simulink model "powertrain"  (R2020b)
settings: Solver=FixedStepAuto  StartTime=0.0  StopTime=t(end)  RelTol=1e-3
PreLoadFcn:
  | C_sc = 1;
StartFcn:
  | C_sc = 1;
values from neighbouring files (symbols this model uses):
  D = 0    [model_fc.m]
  Ts = old_data.Ts    [model_fc.m]
undefined symbols (not defined in the file or in its folder): ANFIS, command, DiscIntNeverNeededParam, ECMS, Flight, in, Ion, Lithium, MPC, out, Tmpc, w
libraries: powerlib x25, neural x25, fuzblock x5, electricdrivelib x3, lib_converters x3, simulink x3, re_lib x1
(part 8 of 8)

== matlab function powertrain/EMS/Management Variant/MPC-1/PV - FC - control ==
  settings: updateMethod=DISCRETE  sampleTime=Ts
  data: Time input; Vdc_command input; Vfc input; Ifc_in input; Vbatt input; Ibatt_in input; Vpv input; Ifc output; Vfc_conv output; IO_fc_conv output; Pload input; Ipv_in input; SOC input; Ipv output; Vpv_conv output; IO_pv_conv output; Ipvout input; Vdc_real input; Pout_real input; Control_pv output; IO_pv_conv_value input; IO_fc_conv_value input; Control_pv_choose_var input
function [Ifc,Vfc_conv,IO_fc_conv,Ipv,Vpv_conv,IO_pv_conv,Control_pv] = fcn(Time, Vdc_command,Vfc,Ifc_in, Vbatt, Ibatt_in, Vpv, Pload, Ipv_in, SOC, Ipvout, Vdc_real, Pout_real, IO_pv_conv_value, IO_fc_conv_value, Control_pv_choose_var)
    
    
    %% Test for pv panel P&O algo
    persistent Ppv_pre Ppv_w_pre;
    dataType = 'double';
    
    if isempty(Ppv_pre)
        Ppv_pre=0;
        Ppv_w_pre = 200;
    end
    
    if Control_pv_choose_var == 0 % Auto
        Control_pv = 2; % 1 = MPPT | 2 = Cascade Control
    else
        Control_pv = Control_pv_choose_var;
    end
    
    % ?? utile pour le début mais ne fonctionne pas après
%         if Pload == 0 && Control_pv_choose_var == 0
%             Control_pv = 1;
%         end
    
    
    
    Ppv_out = Ipvout*Vdc_real;
    Ppv_in = Ipv_in*Vpv;
    Delta_PV = 0.5;
    Ppv_wanted = Ppv_in;
    
    if Control_pv == 2 % Cascade control
        if mod(Time,2e-4) == 0
            if Ppv_in < Ppv_pre
                Ppv_wanted  = Ppv_in - Delta_PV;
            end
            if Ppv_in > Ppv_pre
                Ppv_wanted  = Ppv_in + Delta_PV;
            end
        end
        if Ppv_out < 0
            Ppv_wanted = 180;
        end
        
        Ipv = Ppv_wanted/Vpv;
    else
        Ipv = 0;
    end
%         Ipv = 180/Vpv;
    Vpv_conv = Vdc_command;
    
    
    % PV converter operates ?
    IO_pv_conv = IO_pv_conv_value;
    
    Ppv_pre = Ppv_in;
    Ppv_w_pre = Ppv_wanted;
    
    
    %% Set if needed
    %     Ipv = 185/Vpv;
    
    
    %% Set max current wanted for the fuel cell
    %     Ifc = 200/Vfc; % doesn't work with my own model
    %     Ifc = 7; % doesn't work with battery ??
    Ifc = 1100/Vfc; % work now ??

    Vfc_conv = Vdc_command;
    if Ifc_in < Ifc
        Vfc_conv = 100;
    end

    
    % FC converter operates ?
    IO_fc_conv = IO_fc_conv_value;
    
end

== matlab function powertrain/EMS/Management Variant/ANFIS-ECMS/MATLAB Function ==
  settings: updateMethod=DISCRETE  sampleTime=Ts
  data: Vbatt input; Ibatt input; Ibatt_out input; Ibatt_1 output; Ifc_out input; Vpv input; Ipv input; Ipv_out input; Pload input; Vdc input; Vdc_wanted input; Pout input; Ibatt_2 output; Ibatt_3 output; IO_batt_conv output; IO_batt_conv_value input; Ifc_boost input; Vfc input
function [Ibatt_1, Ibatt_2, Ibatt_3,  IO_batt_conv] = fcn(Vbatt, Ibatt,Ibatt_out, Ifc_out, Vpv, Ipv, Ipv_out,Pload,Vdc,Vdc_wanted, Pout, IO_batt_conv_value, Ifc_boost, Vfc)
    %% Part - 1
    %     FC = Vfc * Ifc_boost;
    %     FC = Vfc * Ifc_in;
    %     FC = Vdc_wanted * Ifc_out;
    FC = Vdc * Ifc_out;
    
    %     PV = Vpv * Ipv_boost;
%         PV = Vpv * Ipv; % stable pv panel but not good
    %     PV = Vdc_wanted * Ipv_out;
    PV = Vdc * Ipv_out; % marche mieux avec celui ci mais pv pas au max
    
    %     Batt = Vbatt * Ibatt;
    Batt = Vdc * Ibatt_out/0.9;
    
    %     Ibatt_1 = (Pload - FC - PV)/Vdc_wanted;
    %     Ibatt_1 = (Pload - FC - PV)/Vdc;
    Ibatt_1 = (Pload - FC - PV - Batt)/Vdc;
    %     Ibatt_1 = -10;
    
    %% Part - 2
    Ibatt_2 = Pload - Pout;
    
    %% Part - 3
    Ibatt_3 = Vdc_wanted - Vdc;
    
    %% Activate conv
    IO_batt_conv = IO_batt_conv_value;
end

== matlab function powertrain/EMS/Management Variant/ANFIS-ECMS/MATLAB Function1 ==
  settings: updateMethod=DISCRETE  sampleTime=Ts
  data: current_comm input; conv output; Pload input; Vbus_required input; current_command output; V_batt_conv output; DV input
function [conv, current_command,V_batt_conv] = fcn(current_comm, Pload, Vbus_required, DV)
    if current_comm < 0
        conv = 1;
        V_batt_conv = Vbus_required; % (55)
    else
        conv = 0;
        V_batt_conv = Vbus_required;
    end
%     V_batt_conv = 120;
    current_command = current_comm;
    Vbatt_conv = V_batt_conv + DV;
end

%     if Pload == 0 || current_comm < 0
%         conv = 1;
%         V_batt_conv = 50;
%     else
%         conv = 0;
%         V_batt_conv = Vbus_required;
%     end
%     current_command = current_comm;

== matlab function powertrain/PEMFC matfunc V3 - multi/MATLAB Function ==
  settings: updateMethod=DISCRETE  sampleTime=Ts
  data: U_H2 output; U_O2 output; R_ohm output; Ifc input; E_Ner output; E_ohm output; E_con output; E_act_steady output; E_act input; E_act_d output; limit output
function [U_H2,U_O2,R_ohm,E_Ner,E_ohm,E_con,E_act_steady,E_act_d,limit] = fcn(Ifc,E_act)
%     https://link.springer.com/article/10.1007/s40565-016-0196-5
%     Modeling and Simulation of a Proton Exchange Membrane Fuel Cell Alongside a Waste Heat Recovery System Based on the Organic Rankine Cycle in MATLAB/SIMULINK Environment
%     MATHEMATICAL MODELLING FOR PROTON EXCHANGE MEMBRANE FUEL CELL (PEMFC) 
%     https://www.scirp.org/pdf/epe_2020112310053180.pdf#page=17&zoom=100,72,604
%     H-Series Fuel Cell Stacks

    %% constants:
    R = 8.3145;
    Pstd = 101325;
    nF = 2*96485;
    C_act = 2;
    A = 19.6*4.0;
    T = 303.15;
    Nfc = 50;
    lambda = 14;
    l = 21e-4 * 10^-2;
%     l = 1.27e-4;
    
    J = Ifc/A;
    JM = 45/A;
    Pa = 1.45;
    Pc = 1;
    Tc = T-273.15;
    coeff = 1;
        
%     if Ifc <=0
%         Ifc = 40;
%     end
    
    PH2Osat = 10^(-2.18+2.95e-2*Tc-9.18e-5*Tc^2+1.44e-7*Tc^3);
    
    P_H2 = 0.5*PH2Osat*(exp(-(1.635*J/T^1.334))*(Pa/PH2Osat)-1);
    P_O2 = PH2Osat*(exp(-(4.192*J/T^1.334))*(Pc/PH2Osat)-1);
    

    %% Saturation at start
    if -1.87e-4*log(Ifc) > 0
        k = 0;
    else
        if -1.87e-4*log(Ifc) < -1.2
            k = -1.2;
        else
            k = -1.87e-4*log(Ifc);
        end
    end
    %% Nernst Voltage
    E_Ner = 1.229 + (T-298.15) * (-0.85e-3) + T*R/nF * log(P_H2*P_O2^0.5);
    
    %% Activation loss
    % Pressure not in Pa ?
    CO2 = (P_O2/(5.08e6))*exp(498/T);
    CH2 = (P_H2/(1.09e6))*exp(-77/T);
    E_act_steady=-0.9514 + T * (2.86e-3+2e-4*log(200)+4.3e-5*log(CH2)+7.4e-5*log(CO2)+k);
%     E_act_steady = -0.9514 + 3.12e-3*T + 7.4e-5*T*log(CO2) -1.87e-4*T*log(Ifc);
    
    %% Ohmic loss
    E_ohm = - Ifc*(l/((lambda*5.139e-3-3.26e-3)*exp(1268*(1/303-1/T))));
    R_ohm = (l/((lambda*5.139e-3-3.26e-3)*exp(1268*(1/303-1/T))));
    
    %% Concentration loss
%     if T>= 312.15
%         E_con = (1.1e-4-1.2e-6*(T-273.15))*exp(8*Ifc/40);
%     else
%         E_con = (3.3e-3-8.2e-5*(T-273.15))*exp(8*Ifc/40);
%     end

%     E_con = 3*R*T/(2*nF)*log(1-J/JM)-1.5607*R*T/(2*nF);
        if J/JM < 1
        E_con = 3*R*T/(2*nF)*log(1-J/JM)-1.5607*R*T/(2*nF);
    else
%         E_con = -abs(3*R*T/(2*nF)*log(complex(1-J/(JM-0.001)))-1.5607*R*T/(2*nF));
        E_con = 3*R*T/(2*nF)*log(J/JM)-1.5607*R*T/(2*nF);
    end
    
    %% with coefficient
    E_con = coeff * E_con;
    E_act_steady = coeff * E_act_steady;
    E_ohm = coeff * E_ohm;
    E_Ner = coeff * E_Ner;
    
        
    %% activation dynamic loss:
    below = -E_act_steady-E_con;
    E_act_d = (Ifc/C_act)*(1-E_act/below);
%     E_act_d = 0;

    %% Fuel utilization
    U_H2 = 60000*Ifc*R*T*Nfc/(nF*1.16*1*0.9995*Pstd);
    
    %% Air utilization
    U_O2 = 60000*Ifc*R*T*Nfc/(2*nF*0.0181*1*0.21*Pstd);
    limit = 1;
    if J/JM >= 1
            E_con = 0;
            E_act_steady = 0;
            E_ohm = 0;
            E_act_d = 0;
            E_Ner = -35*Ifc;
            if E_Ner <= 0
                E_Ner = 0;
            end
            limit = 0;
    end
    
    
    %%
end

== matlab function powertrain/MATLAB Function ==
  settings: updateMethod=DISCRETE  sampleTime=Ts
  data: ep output; ev output; time input; error_power output; Prequired input; Preal input; Vbus_required input; Vbus_real input; error_voltage output
function [ep,ev,error_power, error_voltage] = fcn(time, Prequired, Preal, Vbus_required, Vbus_real)
    ep = (Preal-Prequired)^2;
    ev = (Vbus_real-Vbus_required)^2;
    
    error_power = 100*abs(Preal-Prequired)/abs(Prequired);
    error_voltage = 100*abs(Vbus_real-Vbus_required)/Vbus_required;
end

== matlab function powertrain/EMS/Management Variant/ANFIS-ECMS/PV - FC - control1 ==
  settings: updateMethod=DISCRETE  sampleTime=Ts
  data: Time input; Vdc_command input; Vfc input; Ifc_in input; Vbatt input; Ibatt_in input; Vpv input; Ifc output; Vfc_conv output; IO_fc_conv output; Pload input; Ipv_in input; SOC input; Ipv output; Vpv_conv output; IO_pv_conv output; Ipvout input; Vdc_real input; Pout_real input; Control_pv output; IO_pv_conv_value input; IO_fc_conv_value input; Control_pv_choose_var input; fuzzy_out input; NNres input
function [Ifc,Vfc_conv,IO_fc_conv,Ipv,Vpv_conv,IO_pv_conv,Control_pv] ...
        = fcn(Time, Vdc_command,Vfc,Ifc_in, Vbatt, Ibatt_in, Vpv, Pload,...
        Ipv_in, SOC, Ipvout, Vdc_real, Pout_real, IO_pv_conv_value,...
        IO_fc_conv_value, Control_pv_choose_var, fuzzy_out, NNres)
    
    
    %% PV - Test for pv panel algo in Cascade control
    persistent Ppv_pre Ppv_w_pre;
    dataType = 'double';
    
    if isempty(Ppv_pre)
        Ppv_pre=0;
        Ppv_w_pre = 200;
    end
    
    if Control_pv_choose_var == 0 % Auto
        Control_pv = 2; % 1 = MPPT | 2 = Cascade Control
    else
        Control_pv = Control_pv_choose_var;
    end
    
    % ?? utile pour le début mais ne fonctionne pas après
%         if Pload == 0 && Control_pv_choose_var == 0
%             Control_pv = 1;
%         end
    
    
    
    Ppv_out = Ipvout*Vdc_real;
    Ppv_in = Ipv_in*Vpv;
    Delta_PV = 0.5;
    Ppv_wanted = Ppv_in;
    
    if Control_pv == 2 % Cascade control
        if mod(Time,2e-4) == 0
            if Ppv_in < Ppv_pre
                Ppv_wanted  = Ppv_in - Delta_PV;
            end
            if Ppv_in > Ppv_pre
                Ppv_wanted  = Ppv_in + Delta_PV;
            end
        end
        if Ppv_out < 0
            Ppv_wanted = 180;
        end
        
        Ipv = Ppv_wanted/Vpv;
    else
        Ipv = 0;
    end
    Vpv_conv = Vdc_command;
    
    
    % PV converter operates ?
    IO_pv_conv = IO_pv_conv_value;
    
    Ppv_pre = Ppv_in;
    Ppv_w_pre = Ppv_wanted;
    
    
    
    %% Set current for the FC
    Ifc = fuzzy_out(NNres) * 1100/Vfc;
    

    Vfc_conv = Vdc_command;
    if Ifc_in < Ifc && (Vdc_real > Vdc_command*0.97 || Vdc_real < Vdc_command * 1.03)
        Vfc_conv = 100;
    end
       
    
    % FC converter operates ?
    IO_fc_conv = IO_fc_conv_value;
    
end

== matlab function powertrain/EMS/Management Variant/ECAEMS/MATLAB Function ==
  settings: updateMethod=DISCRETE  sampleTime=Ts
  data: Vbatt input; Ibatt input; Ibatt_out input; Ibatt_1 output; Ifc_out input; Vpv input; Ipv input; Ipv_out input; Pload input; Vdc input; Vdc_wanted input; Pout input; Ibatt_2 output; Ibatt_3 output; IO_batt_conv output; IO_batt_conv_value input; Ifc_boost input; Vfc input
function [Ibatt_1, Ibatt_2, Ibatt_3,  IO_batt_conv] = fcn(Vbatt, Ibatt,Ibatt_out, Ifc_out, Vpv, Ipv, Ipv_out,Pload,Vdc,Vdc_wanted, Pout, IO_batt_conv_value, Ifc_boost, Vfc)
    %% Part - 1
    %     FC = Vfc * Ifc_boost;
    %     FC = Vfc * Ifc_in;
    %     FC = Vdc_wanted * Ifc_out;
    FC = Vdc * Ifc_out;
    
    %     PV = Vpv * Ipv_boost;
%         PV = Vpv * Ipv; % stable pv panel but not good
    %     PV = Vdc_wanted * Ipv_out;
    PV = Vdc * Ipv_out; % marche mieux avec celui ci mais pv pas au max
    
    %     Batt = Vbatt * Ibatt;
    Batt = Vdc * Ibatt_out;
    
    %     Ibatt_1 = (Pload - FC - PV)/Vdc_wanted;
    %     Ibatt_1 = (Pload - FC - PV)/Vdc;
    Ibatt_1 = (Pload - FC - PV - Batt)/Vdc;
    %     Ibatt_1 = -10;
    
    %% Part - 2
    Ibatt_2 = Pload - Pout;
    
    %% Part - 3
    Ibatt_3 = Vdc_wanted - Vdc;
    
    %% Activate conv
    IO_batt_conv = IO_batt_conv_value;
end

== matlab function powertrain/EMS/Management Variant/MPC-1/MATLAB Function2 ==
  settings: updateMethod=DISCRETE  sampleTime=Ts
  data: Vin input; Vin output; Iin output; Iin input; Vdc input; Ifc_out input; Vdc_ref input; ILmax input; time_data input; old_E_act_d input; old_lim input; sampleTime input; Pin output; Vout output; Iout output; Pout output; Ifc_boost output; Tmpc input; IO_fc_conv input; IO_pv_conv input; Control_pv_choose_var input; Vfc_conv output; IO_fc output; Ipv output; Vpv_conv output; IO_pv output; Control_pv output; Pload input; SOC input; Pload_est input; Vdc_command input; Ipv_out input; Pout_real input
function [Vin, Iin, Pin, Vout, Iout, Pout, Ifc_boost, Vfc_conv, IO_fc, ...
        Ipv, Vpv_conv, IO_pv, Control_pv] = test(Vin, Iin, Vdc, Ifc_out,...
        Vdc_ref, ILmax, time_data, old_E_act_d, old_lim, sampleTime,Tmpc, ...
        IO_fc_conv,IO_pv_conv,Control_pv_choose_var, Pload, SOC, ...,
        Pload_est, Vdc_command,Ipv_out, Pout_real)
    
    coder.extrinsic('evalin');
    coder.extrinsic('GlobalSearch');
    coder.extrinsic('createOptimProblem');
    coder.extrinsic('opti_fcn');
    coder.extrinsic('assignin')
    %% init
    persistent data Pfc_command_pre Pload_full Tsss
    
    if isempty(data)
        Pfc_command_pre = 250;
        
        
        
        Pload_full = evalin('base', 'w');
        data = struct;
        %% variables / states
        data.x_k= [-0.014465353509422;72];
        %         [Iin;Vdc];
        data.e_pre = 0;
        data.e2_pre = 0;
        data.pi_pi = 0;
        data.pi_ii = 0;
        data.E_act = 0;
        data.old_E_act_bl = 0;
        data.old_E_act_d = 0;
        data.old_lim = 0;
        data.Efc = Vin;
        
        %% static data
        data.Ts = sampleTime;
        % converter data
        data.L = 2e-3;
        L = 2e-3;
        data.Ca = 1e-4;
        Ca = 1e-4;
        data.Cdc = 1;
        Cdc = 1;
        
        % regulators data
        data.Ct = Ca + Cdc;
        Ct = Ca + Cdc;
        
        T_v_bst = 1;
        T_i_bst = 1;
        damp = 0.707;
        % Current regulator
        zetai=damp;
        thau_si=T_i_bst/10;
        zetawni=(-log(0.05*sqrt(1-zetai^2)))/thau_si;
        data.Kpi=2*L*zetawni / 1000;
        wni=zetawni/zetai;
        data.Kii=L*wni^2 / 1000;
        
        % Voltage regulator
        zetav=damp;
        thau_sv=T_v_bst; %response time
        zetawnv=(-log(0.05*sqrt(1-zetav^2)))/thau_sv;
        data.Kpv=2*Ct*zetawnv;
        wnv=zetawnv/zetav;
        data.Kiv=Ct*wnv^2;
        
        % fuel cell data
        data.Ncell = 50;
        data.eff = 0.9;
        data.T = 303.15;
        data.Rohm = 0.061871;
        data.R_ = 8.3145;
        data.Pstd = 101325;
        data.nF = 2*96485;
        data.C_act = 2;
        A = 19.6*4.0;
        data.A = 19.6*4.0;
        data.Nfc = 50;
        data.lambda = 14;
        data.l = 21e-4 * 10^-2;
        data.JM = 45/A;
        data.Pa = 1.45;
        data.Pc = 1;
        data.coeff = 1;
        Tsss = evalin('base', 'Ts');
    end
    Ts = 1e-3;
    Hp = 20;
    TsOpti = Ts*1e3;
    
    %     Ts = 1e-3; %     Hp = 20; %     TsOpti = Ts*1e3;
    
    
    if Control_pv_choose_var == 0 % Auto
        Control_pv = 2; % 1 = MPPT | 2 = Cascade Control
    else
        Control_pv = Control_pv_choose_var;
    end
    
    IO_pv = IO_pv_conv;
    Vpv_conv = 72;
    Ipv = 0;
    
    
    
    %% approximation of states of the FC part
    %     data.old_E_act_d = old_E_act_d;
    %     data.old_lim = old_lim;
    
    %     data.x_k = [Iin;Vdc];
    
    %     data.Ts = Ts;
    [Vin,Vout,Iout,Pin,Pout,data] = res_fun(Vdc,Ifc_out,ILmax,Vdc_ref,data);
    
    Iin = data.x_k(1);
    Vout = data.x_k(2);
    
    %% FC control
    % FC converter operates ?
    IO_fc = IO_fc_conv;
    
    currind = time_data/Ts;
    
    %     Pload_est = Pload_full(time_data(1)/Ts)
    %     Pload_est = Pload_full(currtime(1:Hp));
    %%%%%%%%
    %%%     ECMS algo:
    %         if (false)
    len = 0;
    len = length(Pload_full);
    if mod((time_data/TsOpti),Hp/2) == 1 && len(1)-currind > TsOpti/Ts*Hp
        SOC_min=40; SOC_max=90;
        Ppv_out = Ipv_out*Vdc;
%         if Pout_real-Ppv_out > 0 || SOC < SOC_min
%             Pfc_command_min=150;
%         else
%             Pfc_command_min = 0;
%         end
        Pfc_command_min=150;
        Pfc_command_max=1100;
        
        size_step = 0:TsOpti/Ts:TsOpti/Ts*Hp;
        currtime = round(currind+size_step);
        Pload_est = Pload_full(currtime(1:Hp));
%         Pload_est = Pload_est - Ppv_out;
        %         Pload_est = sum(Pload_est) - Ppv_out*Hp;
        
        
        
        %define Matrix Aeq
        
        %         Aeq=[0 1];
        %         Aeq=[0 1];
        
        %define Matrix beq
        mu=0.6;
        %         beq=[1-2*mu*((SOC-0.5*(SOC_max+SOC_min))/(SOC_max+SOC_min))];
        k=1-2*mu*((SOC-0.5*(SOC_max+SOC_min))/(SOC_max+SOC_min));
        %     beq=[1-2*mu*((SOC-0.5*(SOC_max+SOC_min))/(SOC_max+SOC_min)); Pload-Ppv_out];
        
        %         %define boundary conditions
        %         lb=[Pfc_command_min, 0];
        %         ub=[Pfc_command_max, 100];
        %
        %         %define initial conditions
        %         x0=[100, 0.1];
        %define boundary conditions
        lb=[Pfc_command_min];
        ub=[Pfc_command_max];
        
        %define initial conditions
        x0=[Pfc_command_pre];
        
        
        %         Pfc_command_pre
        Vdc_real = data.x_k(2);
        Ifc_out = Pout/Vdc_real;
        %         options = optimoptions('fmincon','Algorithm','sqp',...
        %             'Display','off','MaxFunctionEvaluations',500,'MaxIterations',300,...
        %             'DiffMinChange',10);
        %         [y,fval] = fmincon(@(x)loop_res_fun(x,Vin,Vdc,Ifc_out,ILmax,Vdc_ref,data,Hp,Pload_est,k),x0,[],[],[],[],lb,ub,[],options);
        
        Ifc_boost = zeros(1,1);
        y = opti_fcn(x0,lb,ub,Vin,Vdc,Ifc_out,ILmax,Vdc_ref,data,Hp,Pload_est,Ppv_out,k,TsOpti);
        
        Pfc=y(1);
        %         alpha=y(2);
        
        
        %         Pfc = 1100;
    else
        Pfc = Pfc_command_pre;
    end
    Pfc_command_pre = Pfc;
    %%%%%%%%
    
    
    
    Ifc_boost = Pfc/Vin;
    
    % Converter command output voltage
    Vfc_conv = Vdc_command;
    if Iin < Ifc_boost
        %     if Iin < 0.9*Ifc_boost || Iin > 1.1*Ifc_boost
        Vfc_conv = 100;
    end
    
end

% non linear constraints if needed :
% https://fr.mathworks.com/matlabcentral/answers/102632-what-is-the-calling-order-of-the-objective-function-and-nonlinear-constraint-function-for-optimizati

function f = loop_res_fun(x,Vin,Vdc,Ifc_out,ILmax,Vdc_ref,data,Hp,Pload_est,k)
    %     coder.extrinsic('res_fun');
    Ptot_fc = 0;
    err = 0;
    for i=1:Hp
        ILmax = x(1) / Vin;
        Vdc_real = data.x_k(2);
        [Vin,Vout,Iout,Pin,Pout,data] = res_fun(Vdc_real,Ifc_out,ILmax,Vdc_ref,data);
        Vdc_real = data.x_k(2);
        Ifc_out = Pout/Vdc_real;
        if data.x_k(1) > ILmax
            Vdc_ref = 100;
        else
            Vdc_ref = 72;
        end
        Ptot_fc = Ptot_fc + Pin;
        %         if Pload_est(i) - Pout > 850 || Pload_est(i) - Pout < -150
        %             err = err + 1000;
        %         end
    end
    %     f = Hp*data.Ts * (Ptot_fc*(1-x(2)) + x(2)*sum(Pload_est) + err)
    f = Hp*data.Ts * (Ptot_fc*(1-k) + k*sum(Pload_est) + err)
    x
    x-100
    
    
end

function [Vin,Vout,Iout,Pin,Pout,new_data] = res_fun(Vdc,Ifc_out,ILmax,Vdc_ref,data)
    %% get data
    Ts = data.Ts;
    % converter data
    L = data.L;
    Ca = data.Ca;
    
    % Current regulator
    Kpi = data.Kpi;
    Kii = data.Kii;
    
    % Voltage regulator
    Kpv = data.Kpv;
    Kiv = data.Kiv;
    
    % fuel cell data
    Ncell = data.Ncell;
    eff = data.eff;
    T = data.T;
    Rohm = data.Rohm;
    R_ = data.R_;
    Pstd = data.Pstd;
    nF = data.nF;
    C_act = data.C_act;
    Nfc = data.Nfc;
    lambda = data.lambda;
    l = data.l;
    JM = data.JM;
    Pa = data.Pa;
    Pc = data.Pc;
    coeff = data.coeff;
    
    
    
    % states
    %     x_k=[Iin;Vdc];
    x_k=data.x_k;
    e_pre=data.e_pre;
    e2_pre=data.e2_pre;
    pi_pi=data.pi_pi;
    pi_ii=data.pi_ii;
    E_act=data.E_act;
    old_E_act_bl=data.old_E_act_bl;
    old_E_act_d=data.old_E_act_d;
    old_lim=data.old_lim;
    Efc=data.Efc;
    
    
    %% start the function
    R = Vdc/Ifc_out;
    x_k(2) = Vdc; %%%%%%%%%%%% changed here
    
    
    
    % Vdc_ref = given by EMS
    % ILmax = given by EMS
    
    %     if x_k(1)<0.001
    %         x_k(1) = 0.001;
    %     end
    
    
    %     Vin = Efc - Rohm * x_k(1);
    Vin = Efc;
    if Vin <= 0
        Vin = 60.484318707027604;
    end
    
    
    %% BOOST PART
    % control part voltage:
    e=(Vdc_ref - x_k(2));
    %     e=(Vdc_ref - Vdc_real);
    pi_pi = min(0.5,max(-0.5,pi_pi + Kiv*Ts*e_pre)); % sat:[-0.5; 0.5]
    out_pi_1 = min(0.5,max(-0.5,Kpv*e + pi_pi)); % sat:[-0.5; 0.5]
    
    sub = max(0.01,eff*Vin); % sat:[0.01; Inf]
    %     temp = min(ILmax,max(0,(out_pi_1+x_k(2)/R)*x_k(2)/sub)); % sat:[0; ILmax]
    temp = min(ILmax,max(0,(out_pi_1+x_k(2)*(1/(5e3)+1/R))*x_k(2)/sub)); % sat:[0; ILmax]
    %     temp = (out_pi_1+Vdc_real/R)*Vdc_real/sub;
    
    
    % control part current
    e2 = temp - x_k(1);
    %     e2 = temp - iL;
    pi_ii = min(50,max(-50,pi_ii + Kii*Ts*e2_pre)); % sat:[-50; 50]
    out_pi_2 = min(50,max(-50,Kpi*e2 + pi_ii)); % sat:[-50; 50]
    
    sub_2 = max(0.01,x_k(2)); % sat:[0.01; Inf]
    %     sub_2 = max(0.01,Vdc_real);
    d = min(1,max(0,1-(Vin-out_pi_2)/sub_2)); % sat:[0; 1]
    
    
    
    A = [-0.002/L -(1-d)/L;(1-d)*eff/Ca*R/(R+0.002) -1/((R+0.002)*Ca)];
    B = [1/L; 0];
    C = [1 0];
    D = 0;
    
    % continuous to discrete (exact)
    %     Ai = expm(Ts*A);
    %     Bi = inv(A)*(Ai - eye(2))*B;
    
    % approx : (https://en.wikipedia.org/wiki/Discretization)
    Ai = eye(2)+A*Ts;
    Bi = Ts*B;
    
    x_k1 = Ai*x_k+Bi*Vin;
    y = C*x_k;
    
    
    %% Outputs
    x_k = x_k1;
    %     x_k(2) = Vdc_real;
    %     x_k(1) = iL;
    %     if x_k(1) < 0.001
    %         x_k(1) = 0.001;
    %     end
    
    Vout = x_k(2);
    Rreal = R+0.002;
    Iout_1 = Vout/Rreal;
    Iout = (Iout_1 - Vout/(5e3));
    
    % works well
    Vout = 72;
    x_k(2) = Vout;
    
    %     x_k(2) = Vdc;
    Iout = Vout/R;
    
    
    Pin = min(2000,max(-100,  Vin*x_k(1))); % sat:[-100; 2000]
    
    Pout = min(2000,max(-500, Vout*Iout));  % sat:[-500; 2000]
    %     Pout = min(2000,max(-500, 0.9*Pin));  % sat:[-500; 2000]
    
    
    
    %% FC PART
    if x_k(1)<0.001
        x_k(1) = 0.001;
    end
    if x_k(1)>100
        x_k(1) = 100;
    end
    Ifc = x_k(1);
    
    J = Ifc/data.A;
    Tc = T-273.15;
    
    PH2Osat = 10^(-2.18+2.95e-2*Tc-9.18e-5*Tc^2+1.44e-7*Tc^3);
    
    P_H2 = 0.5*PH2Osat*(exp(-(1.635*J/T^1.334))*(Pa/PH2Osat)-1);
    P_O2 = PH2Osat*(exp(-(4.192*J/T^1.334))*(Pc/PH2Osat)-1);
    
    
    % Saturation at start
    if -1.87e-4*log(Ifc) > 0
        k = 0;
    else
        if -1.87e-4*log(Ifc) < -1.2
            k = -1.2;
        else
            k = -1.87e-4*log(Ifc);
        end
    end
    
    % Nernst Voltage
    E_Ner = 1.229 + (T-298.15) * (-0.85e-3) + T*R_/nF * log(P_H2*P_O2^0.5);
    
    % Activation loss
    % Pressure not in Pa ?
    CO2 = (P_O2/(5.08e6))*exp(498/T);
    CH2 = (P_H2/(1.09e6))*exp(-77/T);
    E_act_steady=-0.9514 + T * (2.86e-3+2e-4*log(200)+4.3e-5*log(CH2)+7.4e-5*log(CO2)+k);
    %     E_act_steady = -0.9514 + 3.12e-3*T + 7.4e-5*T*log(CO2) -1.87e-4*T*log(Ifc);
    
    % Ohmic loss
    E_ohm = - Ifc*(l/((lambda*5.139e-3-3.26e-3)*exp(1268*(1/303-1/T))));
    R_ohm = (l/((lambda*5.139e-3-3.26e-3)*exp(1268*(1/303-1/T))));
    
    % Concentration loss
    %     if T>= 312.15
    %         E_con = (1.1e-4-1.2e-6*(T-273.15))*exp(8*Ifc/40);
    %     else
    %         E_con = (3.3e-3-8.2e-5*(T-273.15))*exp(8*Ifc/40);
    %     end
    
    if J/JM < 1
        E_con = 3*R_*T/(2*nF)*log(1-J/JM)-1.5607*R_*T/(2*nF);
    else
        %         E_con = -abs(3*R*T/(2*nF)*log(complex(1-J/(JM-0.001)))-1.5607*R*T/(2*nF));
        E_con = 3*R_*T/(2*nF)*log(J/JM)-1.5607*R_*T/(2*nF);
    end
    
    % with coefficient
    E_con = coeff * E_con;
    E_act_steady = coeff * E_act_steady;
    E_ohm = coeff * E_ohm;
    E_Ner = coeff * E_Ner;
    
    
    % activation dynamic loss:
    below = -E_act_steady-E_con;
    E_act_d = (Ifc/C_act)*(1-E_act/below);
    
    % Fuel utilization
    U_H2 = 60000*Ifc*R_*T*Nfc/(nF*1.16*1*0.9995*Pstd);
    
    % Air utilization
    U_O2 = 60000*Ifc*R_*T*Nfc/(2*nF*0.0181*1*0.21*Pstd);
    limit = 1;
    if J/JM >= 1
        E_con = 0;
        E_act_steady = 0;
        E_ohm = 0;
        E_act_d = 0;
        E_Ner = -35*Ifc;
        if E_Ner <= 0
            E_Ner = 0;
        end
        limit = 0;
    end
    
    
    % Efc
    %     E_act_bl =  (old_E_act_bl + Ts*old_E_act_d);
    E_act_bl =  (old_E_act_bl + Ts*E_act_d);
    old_E_act_d = E_act_d;
    E_act = old_lim *E_act_bl;
    old_lim = limit;
    old_E_act_bl = E_act_bl;
    
%     E_act_bl =  (old_E_act_bl + Ts*old_E_act_d);
%     old_E_act_d = E_act_d;
%     old_E_act_bl = E_act_bl;
%     E_act = old_lim *E_act_bl;
%     old_lim = limit;
    
    old_lim = limit;
    
    Efc = Ncell*(E_Ner + E_ohm + E_con - E_act)-Rohm*x_k(1);
    if Efc <= 0
        Efc = 0;
    end
    %     Vin = Efc;
    Iin = x_k(1);
    
    %% save states + data
    
    data.x_k= x_k;
    data.e_pre =e;
    data.e2_pre = e2;
    data.pi_pi = pi_pi ;
    data.pi_ii = pi_ii ;
    data.E_act = E_act ;
    data.old_E_act_bl = old_E_act_bl ;
    data.old_E_act_d = old_E_act_d;
    data.old_lim = old_lim ;
    data.Efc = Efc;
    
    
    new_data = data;
    
    
    %% compute the new value of limit / E_act / ... based on previous values
end

== matlab function powertrain/EMS/Management Variant/ECAEMS/MATLAB Function1 ==
  settings: updateMethod=DISCRETE  sampleTime=Ts
  data: current_comm input; conv output; Pload input; Vbus_required input; current_command output; V_batt_conv output
function [conv, current_command,V_batt_conv] = fcn(current_comm, Pload, Vbus_required)
    if current_comm < 0
        conv = 1;
        V_batt_conv = Vbus_required; % (55)
    else
        conv = 0;
        V_batt_conv = Vbus_required;
    end
%     V_batt_conv = 120;
    current_command = current_comm;
end

%     if Pload == 0 || current_comm < 0
%         conv = 1;
%         V_batt_conv = 50;
%     else
%         conv = 0;
%         V_batt_conv = Vbus_required;
%     end
%     current_command = current_comm;

== matlab function powertrain/EMS/Management Variant/ECAEMS/PV - FC - control ==
  settings: updateMethod=DISCRETE  sampleTime=Ts
  data: Time input; Vdc_command input; Vfc input; Ifc_in input; Vbatt input; Ibatt_in input; Vpv input; Ifc output; Vfc_conv output; IO_fc_conv output; Pload input; Ipv_in input; SOC input; Ipv output; Vpv_conv output; IO_pv_conv output; Ipvout input; Vdc_real input; Pout_real input; Control_pv output; IO_pv_conv_value input; IO_fc_conv_value input; Control_pv_choose_var input; BATT_SOC input
function [Ifc,Vfc_conv,IO_fc_conv,Ipv,Vpv_conv,IO_pv_conv,Control_pv] = ...
        fcn(Time, Vdc_command,Vfc,Ifc_in, Vbatt, Ibatt_in, Vpv, Pload, ...
        Ipv_in, SOC, Ipvout, Vdc_real, Pout_real, IO_pv_conv_value, ...
        IO_fc_conv_value, Control_pv_choose_var, BATT_SOC)
    
    coder.extrinsic('ECAEMS');
    
%     ECAEMS - Equivalent consumption and expense minimization
%     https://oraprdnt.uqtr.uquebec.ca/pls/public/gscw031?owa_no_site=6410&owa_no_fiche=16&owa_bottin=
    %% PV - MPPT P&O algo in Cascade control
    % Get previous values for the MPPT algo in Cascade control
    persistent Ppv_pre Ppv_w_pre;
    dataType = 'double';
    if isempty(Ppv_pre)
        Ppv_pre=0;
        Ppv_w_pre = 200;
    end
    
    
    % Set the control mode
    if Control_pv_choose_var == 0 % Auto
        Control_pv = 2; % 1 = MPPT | 2 = Cascade Control
    else
        Control_pv = Control_pv_choose_var;
    end
    
    
    Ppv_out = Ipvout*Vdc_real;
    Ppv_in = Ipv_in*Vpv;
    Delta_PV = 0.5;
    Ppv_wanted = Ppv_in;
    
    if Control_pv == 2 % Cascade control
        if mod(Time,2e-4) == 0
            if Ppv_in < Ppv_pre
                Ppv_wanted  = Ppv_in - Delta_PV;
            end
            if Ppv_in > Ppv_pre
                Ppv_wanted  = Ppv_in + Delta_PV;
            end
        end
        if Ppv_out < 0
            Ppv_wanted = 180;
        end
        
        Ipv = Ppv_wanted/Vpv;
    else
        Ipv = 0;
    end
    
    % Converter wanter output voltage
    Vpv_conv = Vdc_command;
    
    
    % PV converter operates ?
    IO_pv_conv = IO_pv_conv_value;
    
    
    % Set the values for the next loop
    Ppv_pre = Ppv_in;
    Ppv_w_pre = Ppv_wanted;
    
    
    
    
    %% FC - control
    % FC converter operates ?
    IO_fc_conv = IO_fc_conv_value;
    
    %% ECAEMS
    Pbatt_min=-150; Pbatt_max=850;
    SOC_min=40; SOC_max=90;
    if Pout_real-Ipvout*Vdc_real > 0 || SOC < SOC_min
        Pfc_min=150;
    else
        Pfc_min = 0;
    end
    Pfc_max=1100; 
    
    %define Matrix Aeq
    Aeq=[0 1 0;1 0 1];
    
    %define Matrix beq
    mu=0.6;
    beq=[1-2*mu*((SOC-0.5*(SOC_max+SOC_min))/(SOC_max+SOC_min)); Pload-Ppv_out];
    
    %define boundary conditions
    lb=[Pfc_min, 0, Pbatt_min];
    ub=[Pfc_max, 100, Pbatt_max];
    
    %define initial conditions
    x0=[1000, 0.1, 500];
    
    options = optimoptions('fmincon','Algorithm','sqp',...
        'Display','off','MaxFunctionEvaluations',500,'MaxIterations',100);
    [y,fval] = fmincon(@(x)decms(x,Vfc,Ifc_in,Ibatt_in,SOC),x0,[],[],Aeq,beq,lb,ub,[],options);
    
    Pfc=y(1); Pbatt=y(3); alpha=y(2);
    
    
    % Ifc command
    Ifc = Pfc/Vfc;
    
    % Converter wanted output voltage
    Vfc_conv = Vdc_command;
    if Ifc_in < Ifc
        Vfc_conv = 100;
    end
    
    
function f = decms(x,Vfc,Ifc_in,Ibatt_in,SOC)
    DT=1e-3;
    do = 0.5e-4;
    do = 1;
    alpha = 4;
    FCcost = 525;
    Hcost = 2;
    BATcost = 640;
    Pfc_nom = 400;
    Q = 15;
    dfc = (do/3600)*(1+alpha/(Pfc_nom^2)*(x(1)-Pfc_nom)^2);
    dbat = (1/Q)*abs(weight_func_1(SOC)*weight_func_2(Ibatt_in)*Ibatt_in);
    mfc_deg = dfc * FCcost / Hcost;
    mbat_deg = dbat * BATcost / Hcost;
%     f = (x(1)+x(2)*x(3)+ mfc_deg + mbat_deg)*DT;
    mfc_deg = dfc * FCcost;
    f = (x(1)+x(2)*x(3)+ mfc_deg)*DT;
%     f = (x(1)*dfc+x(2)*x(3))*DT;
    
function out = weight_func_1(SOC)
    out = 1+3.25*(1-SOC/100)^2;
    
function out = weight_func_2(Ibatt)
    Ibatt_nom = 2;
    if Ibatt >= 0
        out = 1+0.45*Ibatt/Ibatt_nom;
    else
        out = 1+0.55*abs(Ibatt)/Ibatt_nom;
    end

== matlab function powertrain/EMS/Management Variant/SMC/MATLAB Function1 ==
  settings: updateMethod=DISCRETE  sampleTime=Ts
  data: current_comm input; conv output; Pload input; Vbus_required input; current_command output; V_batt_conv output
function [conv, current_command,V_batt_conv] = fcn(current_comm, Pload, Vbus_required)
    if current_comm < 0
        conv = 1;
        V_batt_conv = Vbus_required; % (55)
    else
        conv = 0;
        V_batt_conv = Vbus_required;
    end
%     V_batt_conv = 120;
    current_command = current_comm;
end

%     if Pload == 0 || current_comm < 0
%         conv = 1;
%         V_batt_conv = 50;
%     else
%         conv = 0;
%         V_batt_conv = Vbus_required;
%     end
%     current_command = current_comm;

== matlab function powertrain/PEMFC matfunc/MATLAB Function ==
  data: Ifc input; E output; P_H2 input; P_O2 input; T input; Water_content input; delta_m input; Nfc input; E_Ner output; E_act output; E_ohm output; E_con output; U_H2 output; U_O2 output; Rohm output
function [E,E_Ner,E_act,E_ohm,E_con,U_H2,U_O2,Rohm] = fcn(Ifc,P_H2,P_O2,T,Water_content,delta_m, Nfc)
    R = 8.3145;
    Pstd = 101325;
    nF = 2*96485;
    
%     %% The operating temperature can vary depending on the ambient temp:
%     T = 3+13*exp(0.03*Ta);

    if Ifc <0
        Ifc = 40;
    end
    %% Saturation at start
    if -1.87e-4*log(Ifc) > 0
        k = 0;
    else
        if -1.87e-4*log(Ifc) < -1.2
            k = -1.2;
        else
            k = -1.87e-4*log(Ifc);
        end
    end
    %% Nernst Voltage
    % Pressure not in Pa ?
    E_Ner = 1.229 + (T-298.15) * (-0.85e-3) + T*R/nF * log(P_H2*P_O2^0.5);
    
    %% Activation loss
    % Pressure not in Pa ?
    CO2 = (P_O2/(5.08e6))*exp(498/T);
    CH2 = (P_H2/(1.09e6))*exp(-77/T);
    E_act=-0.9514 + T * (2.86e-3+2e-4*log(200)+4.3e-5*log(CH2)+7.4e-5*log(CO2)+k);
    
    %% Ohmic loss
    E_ohm = - Ifc*(delta_m/((Water_content*5.139e-3-3.26e-3)*exp(1268*(1/303-1/T))));
    
    %% Ohmic resistance
    Rohm = delta_m / (0.005139*Water_content-0.00326)*exp(1268*(1/303-1/T));
    
    %% Concentration loss
    if T>= 312.15
        E_con = (1.1e-4-1.2e-6*(T-273.15))*exp(8*Ifc/40);
    else
        E_con = (3.3e-3-8.2e-5*(T-273.15))*exp(8*Ifc/40);
    end
    
    
    %% Output voltage
    E = Nfc*(E_Ner + E_act + E_ohm - E_con);
    
    
    %% Fuel utilization
    U_H2 = 60000*Ifc*R*T*Nfc/(nF*1.16*1*0.9995*Pstd);
    
    %% Air utilization
    U_O2 = 60000*Ifc*R*T*Nfc/(2*nF*0.0181*1*0.21*Pstd);
end
